simulink model "kp_control"  (R2023a)
settings: Solver=VariableStepAuto  StartTime=0.0  StopTime=10.0  RelTol=1e-3
settings Model: Creator=TUBA  LastModifiedBy=TUBA

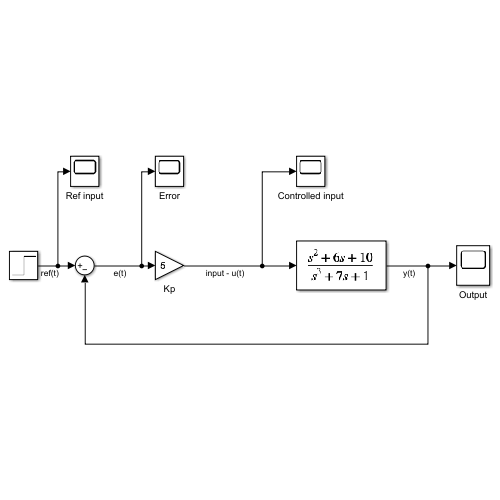
[thumbnail: Simulink's stored preview of the top-level diagram]
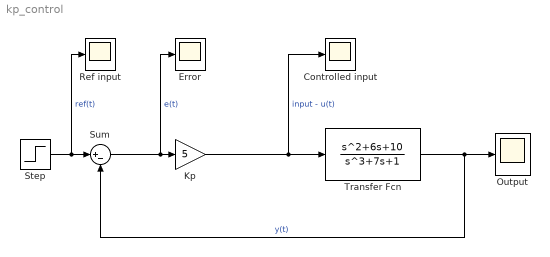
== system kp_control ==
  Controlled input : Scope
  Error : Scope
  Kp : Gain  Gain=5
  Output : Scope
  Ref input : Scope
  Step : Step  SampleTime=0
  Sum : Sum  Inputs=|+-
  Transfer Fcn : TransferFcn  Numerator=[1,6,10]  Denominator=[1,0,7,1]
  wires:
  Transfer Fcn/1 -> Output/1, Sum/2  "y(t)"
  Step/1 -> Ref input/1, Sum/1  "ref(t)"
  Sum/1 -> Error/1, Kp/1  "e(t)"
  Kp/1 -> Controlled input/1, Transfer Fcn/1  "input - u(t)"
